simulink model "PumpModel"  (R2017b)
settings: Solver=VariableStepAuto  StartTime=0.0  StopTime=10  RelTol=1e-3
libraries: simulink x2
settings Model: Creator=db217620  LastModifiedBy=db217620
settings SolverCC: AlgebraicLoopSolver=LineSearch

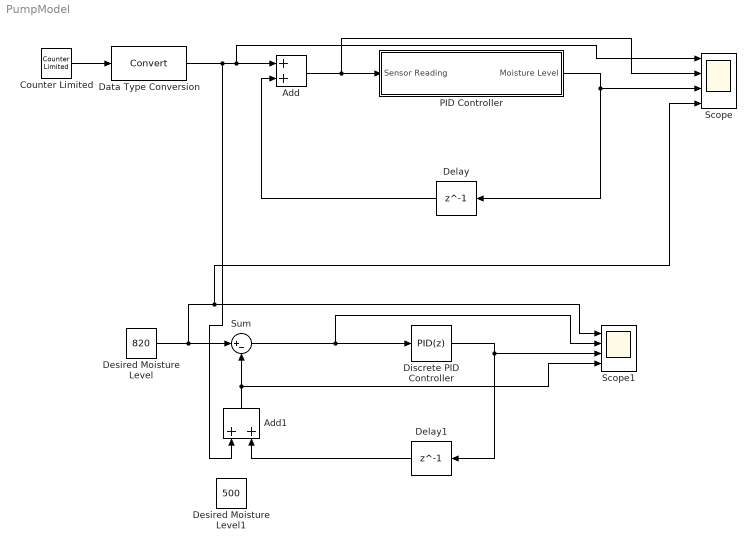
== system PumpModel ==
  Add : Sum
  Add1 : Sum
  Counter Limited : simulink/Sources/Counter Limited  uplimit=1023  tsamp=.01
  Data Type Conversion : DataTypeConversion
  Delay : Delay  DelayLength=1  InitialCondition=0
  Delay1 : Delay  DelayLength=1  InitialCondition=0
  Desired Moisture Level : Constant  Value=820
  Desired Moisture Level1 : Constant  Value=500
  Discrete PID Controller : simulink/Continuous/PID Controller  Controller=PID  TimeDomain=Discrete-time  SampleTime=-1  IntegratorMethod=Forward Euler  FilterMethod=Forward Euler  Form=Parallel  UseFilter=off  ControllerParametersSource=internal  P=.6  I=5  D=0  N=100  InitialConditionSource=internal  InitialConditionForIntegrator=0  InitialConditionForFilter=0  ExternalReset=none  LimitOutput=off  UpperSaturationLimit=inf  LowerSaturationLimit=-inf  LinearizeAsGain=off  AntiWindupMode=none  Kb=1  TrackingMode=off  Kt=1  PParamMin=[]  PParamMax=[]  IParamMin=[]  IParamMax=[]  DParamMin=[]  DParamMax=[]  NParamMin=[]  NParamMax=[]  KbParamMin=[]  KbParamMax=[]  KtParamMin=[]  KtParamMax=[]  POutMin=[]  POutMax=[]  IOutMin=[]  IOutMax=[]  DOutMin=[]  DOutMax=[]  NOutMin=[]  NOutMax=[]  KbOutMin=[]  KbOutMax=[]  KtOutMin=[]  KtOutMax=[]  IntegratorOutMin=[]  IntegratorOutMax=[]  FilterOutMin=[]  FilterOutMax=[]  SumOutMin=[]  SumOutMax=[]  SumI1OutMin=[]  SumI1OutMax=[]  SumI2OutMin=[]  SumI2OutMax=[]  SumI3OutMin=[]  SumI3OutMax=[]  SumDOutMin=[]  SumDOutMax=[]  SaturationOutMin=[]  SaturationOutMax=[]  IntegratorContinuousStateAttributes=''  IntegratorStateMustResolveToSignalObject=off  IntegratorRTWStateStorageClass=Auto  FilterContinuousStateAttributes=''  FilterStateMustResolveToSignalObject=off  FilterRTWStateStorageClass=Auto  DifferentiatorICPrevScaledInput=0  DifferentiatorOutMin=[]  DifferentiatorOutMax=[]  InitialConditionSetting=State (most efficient)  FilterDiffOutCoefMin=[]  FilterDiffOutCoefMax=[]  SumDenOutMin=[]  SumDenOutMax=[]  SumNumOutMin=[]  SumNumOutMax=[]  ReciprocalOutMin=[]  ReciprocalOutMax=[]  DivideOutMin=[]  DivideOutMax=[]  TunerSelectOption=Transfer Function Based (PID Tuner App)
  PID Controller : Subsystem
  Scope : Scope  NumInputPorts=4
  Scope1 : Scope  NumInputPorts=4
  Sum : Sum  Inputs=|+-
  wires:
  Counter Limited/1 -> Data Type Conversion/1
  Data Type Conversion/1 -> Add1/1, Scope/1, Add/1
  Add/1 -> Scope/2, PID Controller/1(Sensor Reading)
  PID Controller/1(Moisture Level) -> Delay/1, Scope/3
  Delay/1 -> Add/2
  Sum/1 -> Scope1/2, Discrete PID Controller/1
  Discrete PID Controller/1 -> Scope1/3, Delay1/1
  Desired Moisture Level/1 -> Scope/4, Scope1/1, Sum/1
  Add1/1 -> Scope1/4, Sum/2
  Delay1/1 -> Add1/2

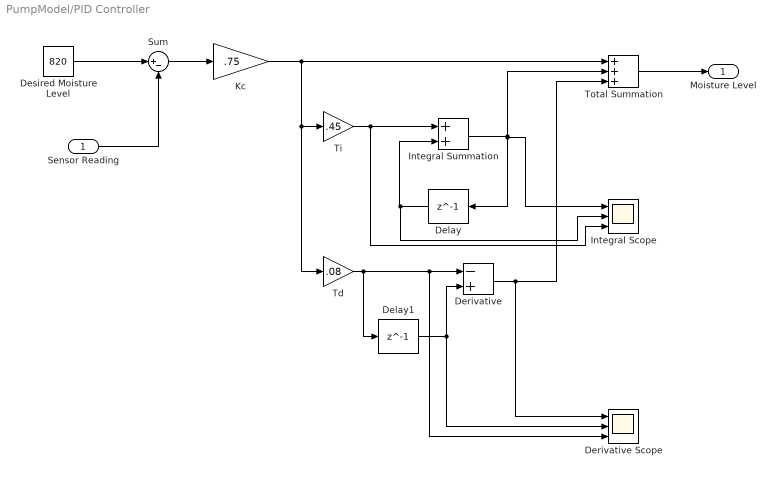
== system PumpModel/PID Controller ==
  Sensor Reading : Inport
  Delay : Delay  DelayLength=1  InitialCondition=0
  Delay1 : Delay  DelayLength=1  InitialCondition=0
  Derivative : Sum  Inputs=-+
  Derivative Scope : Scope  NumInputPorts=3
  Desired Moisture Level : Constant  Value=820
  Integral Scope : Scope  NumInputPorts=3
  Integral Summation : Sum
  Kc : Gain  Gain=.75
  Sum : Sum  Inputs=|+-
  Td : Gain  Gain=.08
  Ti : Gain  Gain=.45
  Total Summation : Sum  Inputs=+++
  Moisture Level : Outport
  wires:
  Desired Moisture Level/1 -> Sum/1
  Sensor Reading/1 -> Sum/2
  Sum/1 -> Kc/1
  Kc/1 -> Ti/1, Td/1, Total Summation/1
  Ti/1 -> Integral Scope/3, Integral Summation/1
  Integral Summation/1 -> Total Summation/2, Integral Scope/1, Delay/1
  Total Summation/1 -> Moisture Level/1
  Delay/1 -> Integral Scope/2, Integral Summation/2
  Td/1 -> Derivative Scope/3, Derivative/1, Delay1/1
  Delay1/1 -> Derivative Scope/2, Derivative/2
  Derivative/1 -> Derivative Scope/1, Total Summation/3
